simulink model "sim3"  (R2018a)
settings: Solver=ode4  StartTime=0.0  StopTime=10.0  FixedStep=0.01  RelTol=1e-3
values from neighbouring files (symbols this model uses):
  A = P * J / P    [s2.m]    (also in s3.m = [0,1;-4,-4]; script.m = nyquist(G1))
  Adys = expm(h*A)    [s3.m]
  B = [1;0]    [s3.m]    (also in script.m = nyquist(G2))
  Bdys = double( int(expm(s*A)*B,s,0,h))    [s3.m]
  C = 0.1    [s1.m]    (also in s3.m = [1, 0; 0, 1])
  Cdys = C    [s3.m]
  D = zeros(size(B))    [s3.m]
  h = 1    [s3.m]
  WPC = 4    [s1.m]    (also in s2.m = WPCa(:,:,2); s3.m = 1000)
settings Model: Creator=Aleksander  LastModifiedBy=Igor
settings DataIOCC: SaveFormat=Array
settings OptimizationCC: LifeSpan=inf
settings DebuggingCC: UnderspecifiedInitializationDetection=Classic  MergeDetectMultiDrivingBlocksExec=none  MultiTaskDSMMsg=warning  MultiTaskCondExecSysMsg=none  FcnCallInpInsideContextMsg=warning  StateNameClashWarn=warning  SFUnexpectedBacktrackingDiag=warning  SFNoUnconditionalDefaultTransitionDiag=warning  SFExecutionAtInitializationDiag=none
settings HardwareCC: ProdBitPerPointer=32  ProdBitPerSizeT=32  ProdBitPerPtrDiffT=32  ProdLargestAtomicFloat=None  ProdIntDivRoundTo=Undefined  ProdEndianess=Unspecified  ProdWordSize=32  ProdHWDeviceType=32-bit Generic
settings ModelReferenceCC: PropagateSignalLabelsOutOfModel=off
settings CodeAppCC: StateflowObjectComments=on
settings GRTTargetCC: TargetLangStandard=C89/C90 (ANSI)  GeneratePreprocessorConditionals=Disable all
settings ConfigComp: CovMetricSettings=dw  CovHtmlReporting=on  CovSaveCumulativeToWorkspaceVar=on  CovSaveSingleToWorkspaceVar=on  CovExternalEMLEnable=off

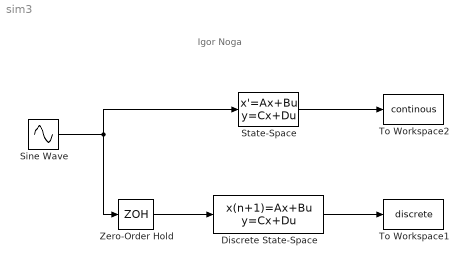
== system sim3 ==
  note: Igor Noga
  Discrete State-Space : DiscreteStateSpace  A=Adys  B=Bdys  C=Cdys  D=D  InitialCondition=WPC
  Sine Wave : Sin  SampleTime=0
  State-Space : StateSpace  A=A  B=B  C=C  D=D  InitialCondition=WPC
  To Workspace1 : ToWorkspace  VariableName=discrete  SampleTime=-1
  To Workspace2 : ToWorkspace  VariableName=continous  SaveFormat=Timeseries  SampleTime=-1
  Zero-Order Hold : ZeroOrderHold  SampleTime=h
  wires:
  Zero-Order Hold/1 -> Discrete State-Space/1
  State-Space/1 -> To Workspace2/1
  Sine Wave/1 -> Zero-Order Hold/1, State-Space/1
  Discrete State-Space/1 -> To Workspace1/1
